simulink model "redundancy_controller_simulink"  (Simulink 7.5)
settings: Solver=ode45  StartTime=0.0  StopTime=10.0  RelTol=1e-3
settings Model: Creator=konstantinos  LastModifiedBy=konstantinos

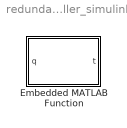
== system redundancy_controller_simulink ==
  Embedded MATLAB Function : Stateflow chart  TreatAsAtomicUnit=on

== matlab function Embedded MATLAB Function ==
  data: q input double; t output double
%#eml
function t = redundancy_controller(q)


K_P=50;

a=1;
tau = zeros(1,16);

for i=1:4:16
    tau(i:i+3) = (K_P*(q(i+2)-a*q(i+3)))*[0 0 1 -1];
end

t=tau;
% t=(eye(16)-JH'*JH)*tau';

% size(JH')
% size(pinv(JH')*JH')
% size(tau')
